simulink model "complete_model MEMBRANA_CALAMAR_GIGANTE_2B"  (R2021a)
settings: Solver=FixedStepAuto  StartTime=0.0  StopTime=30e-3  FixedStep=30e-6  RelTol=1e-3  EnableMultiTasking=on
undefined symbols (not defined in the file or in its folder): Mag_pulso_corriente
settings Model: Creator=ELETRONICA  LastModifiedBy=Bremdows
settings SolverCC: AlgebraicLoopSolver=TrustRegion
settings DataIOCC: LimitDataPoints=on  SaveFormat=Array  SignalLoggingSaveFormat=ModelDataLogs  ReturnWorkspaceOutputs=off
settings OptimizationCC: BlockReduction=off  BooleanDataType=off  BufferReuse=off  ExpressionDepthLimit=2147483647  InitFltsAndDblsToZero=on  LifeSpan=inf
settings DebuggingCC: SaveWithParameterizedLinksMsg=none  UnderspecifiedInitializationDetection=Classic  MergeDetectMultiDrivingBlocksExec=none  SignalResolutionControl=TryResolveAllWithWarning  MultiTaskDSMMsg=warning  MultiTaskCondExecSysMsg=none  FcnCallInpInsideContextMsg=warning  StateNameClashWarn=warning  SFUnexpectedBacktrackingDiag=warning  SFNoUnconditionalDefaultTransitionDiag=warning  SFExecutionAtInitializationDiag=none  SFMachineParentedDataDiag=warning  ArithmeticOperatorsInVariantConditions=warning
settings HardwareCC: ProdBitPerPointer=32  ProdBitPerSizeT=32  ProdBitPerPtrDiffT=32  ProdLargestAtomicFloat=None  ProdIntDivRoundTo=Undefined  ProdEndianess=Unspecified  ProdWordSize=32  ProdHWDeviceType=32-bit Generic  TargetUnknown=on
settings ModelReferenceCC: PropagateSignalLabelsOutOfModel=off
settings SFSimCC: SimUseLocalCustomCode=off  CustomCodeUndefinedFunction=UseInterfaceOnly
settings RTWCC: Description=Generic Real-Time Target  RTWUseLocalCustomCode=off
settings CodeAppCC: StateflowObjectComments=on
settings GRTTargetCC: TargetFcnLib=ansi_tfl_tmw.mat  TargetLangStandard=C89/C90 (ANSI)  CombineOutputUpdateFcns=off  GRTInterface=on
settings ConfigComp: CovMetricSettings=dw  CovSaveCumulativeToWorkspaceVar=on  CovSaveSingleToWorkspaceVar=on  CovExternalEMLEnable=off

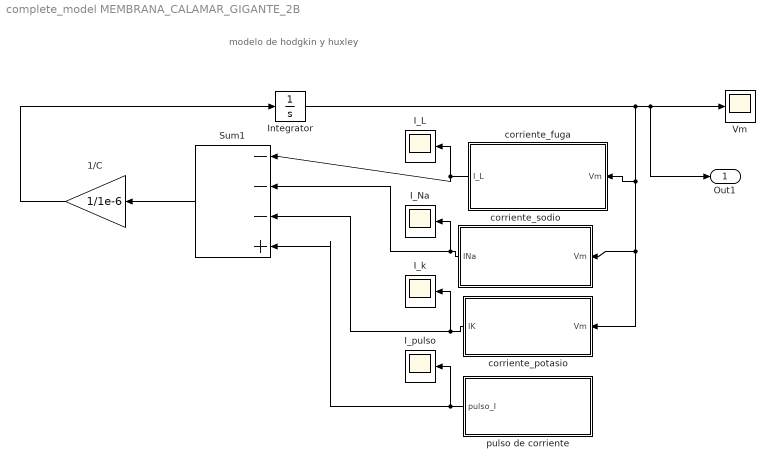
== system complete_model MEMBRANA_CALAMAR_GIGANTE_2B ==
  note: modelo de hodgkin y huxley
  1/C : Gain  Gain=1/1e-6  SaturateOnIntegerOverflow=on  OutDataTypeStr=Inherit: Same as input  ParamDataTypeStr=Inherit: Same as input
  I_L : Scope
  I_Na : Scope
  I_k : Scope
  I_pulso : Scope
  Integrator : Integrator  InitialCondition=-60e-3
  Sum1 : Sum  Inputs=|---+  SaturateOnIntegerOverflow=on
  Vm : Scope
  corriente_fuga : Subsystem
  corriente_potasio : Subsystem
  corriente_sodio : Subsystem
  pulso de corriente : Subsystem
  Out1 : Outport  VectorParamsAs1DForOutWhenUnconnected=off
  wires:
  Sum1/1 -> 1/C/1
  corriente_potasio/1(IK) -> I_k/1, Sum1/3
  corriente_sodio/1(INa) -> Sum1/2, I_Na/1
  corriente_fuga/1(I_L) -> Sum1/1, I_L/1
  1/C/1 -> Integrator/1
  Integrator/1 -> corriente_potasio/1(Vm), corriente_sodio/1(Vm), corriente_fuga/1(Vm), Vm/1, Out1/1
  pulso de corriente/1(pulso_I) -> Sum1/4, I_pulso/1

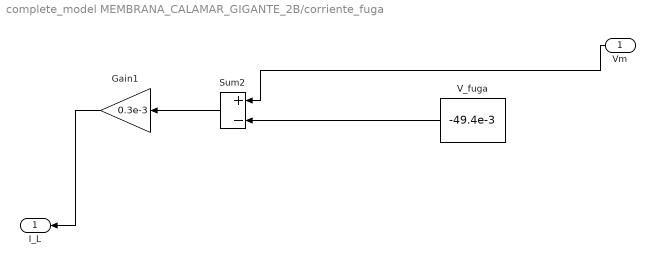
== system complete_model MEMBRANA_CALAMAR_GIGANTE_2B/corriente_fuga ==
  Vm : Inport
  Gain1 : Gain  Gain=0.3e-3  SaturateOnIntegerOverflow=on  OutDataTypeStr=Inherit: Same as input  ParamDataTypeStr=Inherit: Same as input
  Sum2 : Sum  Inputs=|+-  SaturateOnIntegerOverflow=on
  V_fuga : Constant  Value=-49.4e-3
  I_L : Outport  VectorParamsAs1DForOutWhenUnconnected=off
  wires:
  Sum2/1 -> Gain1/1
  V_fuga/1 -> Sum2/2
  Vm/1 -> Sum2/1
  Gain1/1 -> I_L/1

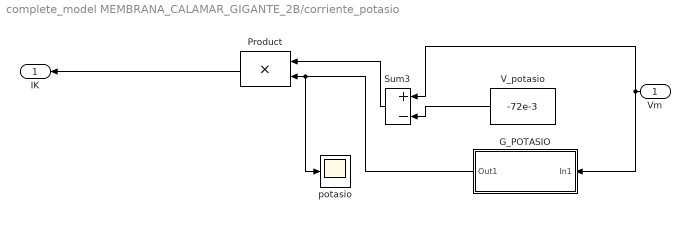
== system complete_model MEMBRANA_CALAMAR_GIGANTE_2B/corriente_potasio ==
  Vm : Inport
  G_POTASIO : Subsystem
  Product : Product  SaturateOnIntegerOverflow=on  OutDataTypeStr=Inherit: Same as first input
  Sum3 : Sum  Inputs=|+-  SaturateOnIntegerOverflow=on
  V_potasio : Constant  Value=-72e-3
  potasio : Scope
  IK : Outport  VectorParamsAs1DForOutWhenUnconnected=off
  wires:
  Sum3/1 -> Product/1
  V_potasio/1 -> Sum3/2
  G_POTASIO/1(Out1) -> Product/2, potasio/1
  Vm/1 -> Sum3/1, G_POTASIO/1(In1)
  Product/1 -> IK/1

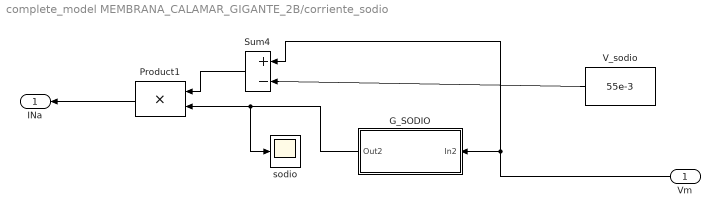
== system complete_model MEMBRANA_CALAMAR_GIGANTE_2B/corriente_sodio ==
  Vm : Inport
  G_SODIO : Subsystem
  Product1 : Product  SaturateOnIntegerOverflow=on  OutDataTypeStr=Inherit: Same as first input
  Sum4 : Sum  Inputs=|+-  SaturateOnIntegerOverflow=on
  V_sodio : Constant  Value=55e-3
  sodio : Scope
  INa : Outport  VectorParamsAs1DForOutWhenUnconnected=off
  wires:
  Sum4/1 -> Product1/1
  V_sodio/1 -> Sum4/2
  G_SODIO/1(Out2) -> Product1/2, sodio/1
  Vm/1 -> Sum4/1, G_SODIO/1(In2)
  Product1/1 -> INa/1

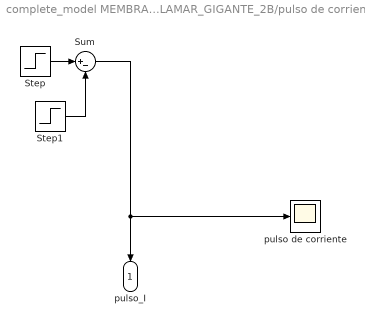
== system complete_model MEMBRANA_CALAMAR_GIGANTE_2B/pulso de corriente ==
  Step : Step  Time=1e-3  After=Mag_pulso_corriente  SampleTime=0  VectorParams1D=off
  Step1 : Step  Time=2e-3  After=Mag_pulso_corriente  SampleTime=0  VectorParams1D=off
  Sum : Sum  Inputs=|+-  SaturateOnIntegerOverflow=on
  pulso de corriente : Scope
  pulso_I : Outport  VectorParamsAs1DForOutWhenUnconnected=off
  wires:
  Step/1 -> Sum/1
  Step1/1 -> Sum/2
  Sum/1 -> pulso de corriente/1, pulso_I/1

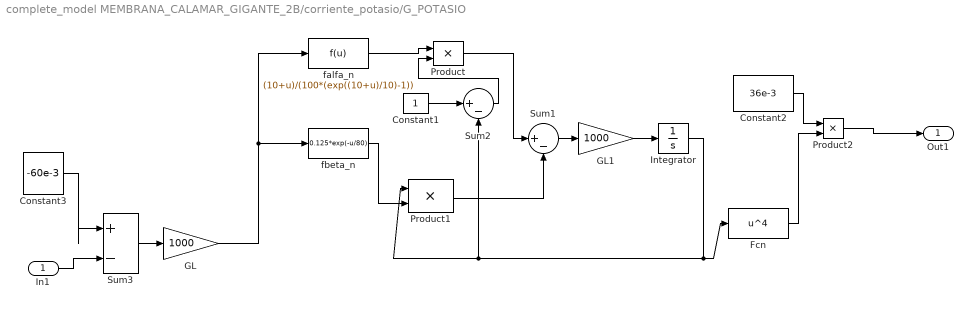
== system complete_model MEMBRANA_CALAMAR_GIGANTE_2B/corriente_potasio/G_POTASIO ==
  In1 : Inport
  Constant1 : Constant
  Constant2 : Constant  Value=36e-3  VectorParams1D=off
  Constant3 : Constant  Value=-60e-3
  Fcn : Fcn  Expr=u^4
  GL : Gain  Gain=1000  SaturateOnIntegerOverflow=on  OutDataTypeStr=Inherit: Same as input  ParamDataTypeStr=Inherit: Same as input
  GL1 : Gain  Gain=1000  SaturateOnIntegerOverflow=on  OutDataTypeStr=Inherit: Same as input  ParamDataTypeStr=Inherit: Same as input
  Integrator : Integrator  InitialCondition=0.317
  Product : Product  SaturateOnIntegerOverflow=on  OutDataTypeStr=Inherit: Same as first input
  Product1 : Product  SaturateOnIntegerOverflow=on  OutDataTypeStr=Inherit: Same as first input
  Product2 : Product  SaturateOnIntegerOverflow=on  OutDataTypeStr=Inherit: Same as first input
  Sum1 : Sum  Inputs=|+-  SaturateOnIntegerOverflow=on
  Sum2 : Sum  Inputs=|+-  SaturateOnIntegerOverflow=on
  Sum3 : Sum  Inputs=|+-  SaturateOnIntegerOverflow=on
  falfa_n : Fcn  Expr=(10+u)/(100*(exp((10+u)/10)-1))
  fbeta_n : Fcn  Expr=0.125*exp(-u/80)
  Out1 : Outport  VectorParamsAs1DForOutWhenUnconnected=off
  wires:
  falfa_n/1 -> Product/1
  fbeta_n/1 -> Product1/2
  Fcn/1 -> Product2/2
  Constant2/1 -> Product2/1
  Product2/1 -> Out1/1
  Constant1/1 -> Sum2/1
  Sum2/1 -> Product/2
  Integrator/1 -> Sum2/2, Product1/1, Fcn/1
  Product/1 -> Sum1/1
  Product1/1 -> Sum1/2
  Sum1/1 -> GL1/1
  Sum3/1 -> GL/1
  GL/1 -> falfa_n/1, fbeta_n/1
  GL1/1 -> Integrator/1
  Constant3/1 -> Sum3/1
  In1/1 -> Sum3/2

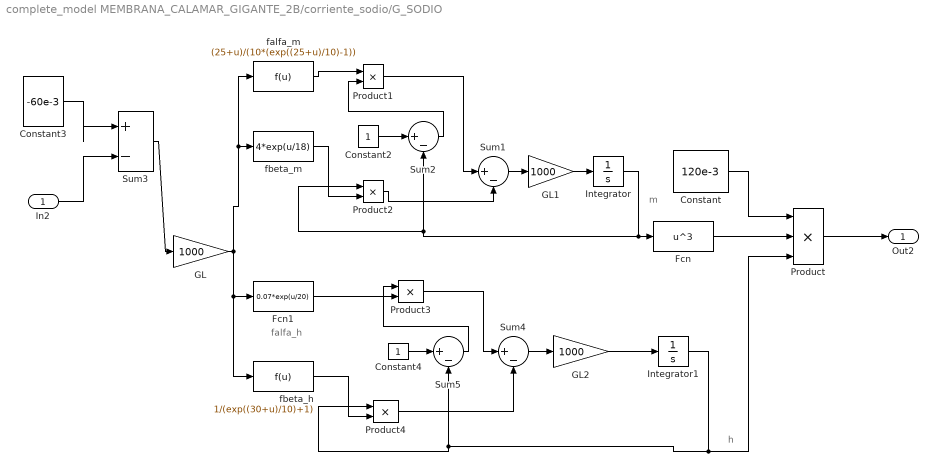
== system complete_model MEMBRANA_CALAMAR_GIGANTE_2B/corriente_sodio/G_SODIO ==
  note: falfa_h
  note: m
  note: h
  In2 : Inport
  Constant : Constant  Value=120e-3
  Constant2 : Constant
  Constant3 : Constant  Value=-60e-3
  Constant4 : Constant
  Fcn : Fcn  Expr=u^3
  Fcn1 : Fcn  Expr=0.07*exp(u/20)
  GL : Gain  Gain=1000  SaturateOnIntegerOverflow=on  OutDataTypeStr=Inherit: Same as input  ParamDataTypeStr=Inherit: Same as input
  GL1 : Gain  Gain=1000  SaturateOnIntegerOverflow=on  OutDataTypeStr=Inherit: Same as input  ParamDataTypeStr=Inherit: Same as input
  GL2 : Gain  Gain=1000  SaturateOnIntegerOverflow=on  OutDataTypeStr=Inherit: Same as input  ParamDataTypeStr=Inherit: Same as input
  Integrator : Integrator  InitialCondition=0.053
  Integrator1 : Integrator  InitialCondition=0.596
  Product : Product  Inputs=3  RndMeth=Zero
  Product{1..4} (4 alike) : Product  SaturateOnIntegerOverflow=on  OutDataTypeStr=Inherit: Same as first input
  Sum{1..5} (5 alike) : Sum  Inputs=|+-  SaturateOnIntegerOverflow=on
  falfa_m : Fcn  Expr=(25+u)/(10*(exp((25+u)/10)-1))
  fbeta_h : Fcn  Expr=1/(exp((30+u)/10)+1)
  fbeta_m : Fcn  Expr=4*exp(u/18)
  Out2 : Outport  VectorParamsAs1DForOutWhenUnconnected=off
  wires:
  Constant/1 -> Product/1
  Fcn/1 -> Product/2
  falfa_m/1 -> Product1/1
  fbeta_m/1 -> Product2/2
  Constant2/1 -> Sum2/1
  Sum2/1 -> Product1/2
  Product1/1 -> Sum1/1
  Product2/1 -> Sum1/2
  Sum1/1 -> GL1/1
  Integrator/1 -> Sum2/2, Product2/1, Fcn/1
  Fcn1/1 -> Product3/1
  fbeta_h/1 -> Product4/2
  Constant4/1 -> Sum5/1
  Sum5/1 -> Product3/2
  Integrator1/1 -> Product4/1, Sum5/2, Product/3
  Product3/1 -> Sum4/1
  Product4/1 -> Sum4/2
  Sum4/1 -> GL2/1
  Product/1 -> Out2/1
  Sum3/1 -> GL/1
  GL/1 -> falfa_m/1, fbeta_m/1, Fcn1/1, fbeta_h/1
  GL1/1 -> Integrator/1
  GL2/1 -> Integrator1/1
  Constant3/1 -> Sum3/1
  In2/1 -> Sum3/2
